simulink model "gm_uz_plantModel_pt1"  (R2020b)
settings: Solver=FixedStepAuto  StartTime=0.0  StopTime=20  RelTol=1e-3
libraries: dspsigops x11, hdlmdlgenlib x6
settings Model: Creator=ts  LastModifiedBy=ts
settings DataIOCC: LimitDataPoints=on  SaveOutput=off  SaveTime=off
settings OptimizationCC: BlockReduction=off  ConditionallyExecuteInputs=off  DefaultParameterBehavior=Inlined  LifeSpan=inf
settings DebuggingCC: AlgebraicLoopMsg=error  InheritedTsInSrcMsg=none  SingleTaskRateTransMsg=error  AllowSymbolicDim=off  StrictBusMsg=ErrorOnBusTreatedAsVector  SFUnexpectedBacktrackingDiag=warning  SFNoUnconditionalDefaultTransitionDiag=warning  SFExecutionAtInitializationDiag=none  ArithmeticOperatorsInVariantConditions=warning
settings HardwareCC: ProdBitPerPointer=32  ProdBitPerSizeT=32  ProdBitPerPtrDiffT=32  ProdLargestAtomicFloat=None  ProdIntDivRoundTo=Undefined  ProdEndianess=Unspecified  ProdWordSize=32  ProdHWDeviceType=ASIC/FPGA->ASIC/FPGA  ProdEqTarget=off
settings SFSimCC: SimUseLocalCustomCode=off  CustomCodeUndefinedFunction=UseInterfaceOnly
settings RTWCC: RTWUseLocalCustomCode=off
settings CodeAppCC: StateflowObjectComments=on
settings GRTTargetCC: TargetLangStandard=C89/C90 (ANSI)
settings ConfigComp: CovScope=ReferencedModels  CovMetricSettings=dw  CovSaveCumulativeToWorkspaceVar=on  CovSaveSingleToWorkspaceVar=on  CovExternalEMLEnable=off  CovSFcnEnable=off

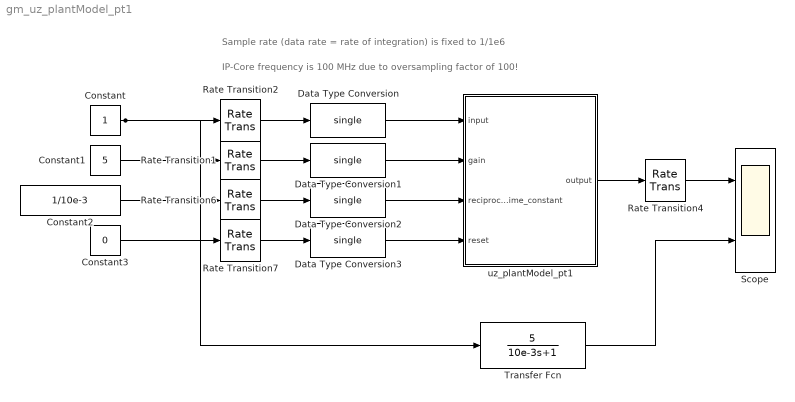
== system gm_uz_plantModel_pt1 ==
  note: Sample rate (data rate = rate of integration) is fixed to 1/1e6
  note: IP-Core frequency is 100 MHz due to oversampling factor of 100!
  Constant : Constant
  Constant1 : Constant  Value=5
  Constant2 : Constant  Value=1/10e-3
  Constant3 : Constant  Value=0
  Data Type Conversion{,1..3} (4 alike) : DataTypeConversion  OutDataTypeStr=single
  Rate Transition{1..2,6..7} (4 alike) : RateTransition  OutPortSampleTime=1/1e6
  Rate Transition4 : RateTransition
  Scope : Scope  NumInputPorts=2
  Transfer Fcn : TransferFcn  Numerator=[5]  Denominator=[10e-3 1]
  uz_plantModel_pt1 : Subsystem  TreatAsAtomicUnit=on
  wires:
  Constant3/1 -> Rate Transition7/1
  Constant2/1 -> Rate Transition6/1
  Constant1/1 -> Rate Transition1/1
  Rate Transition7/1 -> Data Type Conversion3/1
  Rate Transition6/1 -> Data Type Conversion2/1
  Rate Transition1/1 -> Data Type Conversion1/1
  Data Type Conversion3/1 -> uz_plantModel_pt1/4(reset)
  Data Type Conversion2/1 -> uz_plantModel_pt1/3(reciprocal_time_constant)
  Data Type Conversion1/1 -> uz_plantModel_pt1/2(gain)
  Data Type Conversion/1 -> uz_plantModel_pt1/1(input)
  Rate Transition2/1 -> Data Type Conversion/1
  Transfer Fcn/1 -> Scope/2
  Rate Transition4/1 -> Scope/1
  Constant/1 -> Transfer Fcn/1, Rate Transition2/1
  uz_plantModel_pt1/1(output) -> Rate Transition4/1

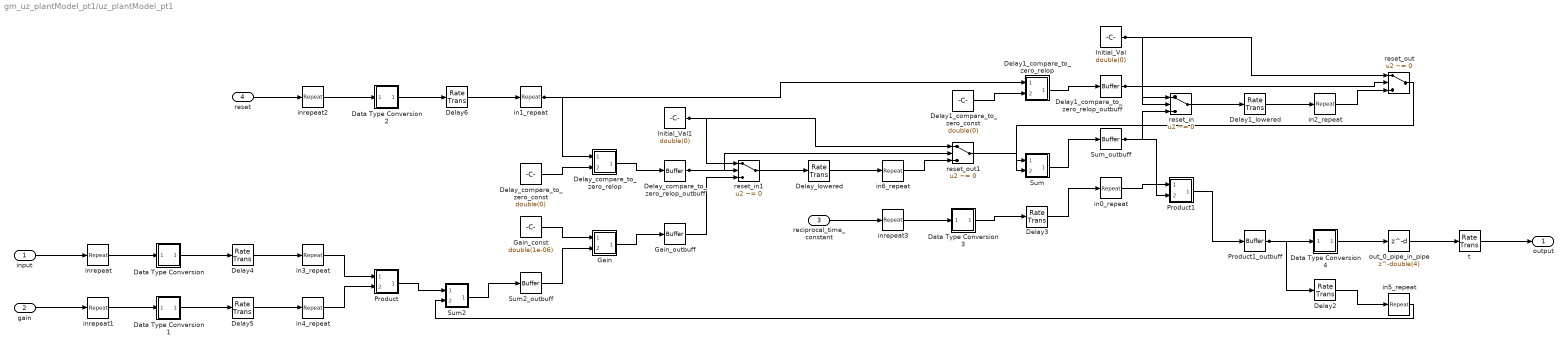
== system gm_uz_plantModel_pt1/uz_plantModel_pt1 ==
  input : Inport  OutDataTypeStr=single  PortDimensions=1  SampleTime=1e-06
  gain : Inport  Port=2  OutDataTypeStr=single  PortDimensions=1  SampleTime=1e-06
  reciprocal_time_constant : Inport  Port=3  OutDataTypeStr=single  PortDimensions=1  SampleTime=1e-06
  reset : Inport  Port=4  OutDataTypeStr=single  PortDimensions=1  SampleTime=1e-06
  Data Type Conversion : Subsystem
      mask Display: disp('NFP\nconv');
  Data Type Conversion1 : Subsystem
      mask Display: disp('NFP\nconv');
  Data Type Conversion2 : Subsystem
      mask Display: disp('NFP\nconv');
  Data Type Conversion3 : Subsystem
      mask Display: disp('NFP\nconv');
  Data Type Conversion4 : Subsystem
      mask Display: disp('NFP\nconv');
  Delay1_compare_to_zero_const : Constant  Value=double(0)  OutDataTypeStr=double  SampleTime=1e-08
  Delay1_compare_to_zero_relop : Subsystem
      mask Display: disp('NFP\nrelop');
  Delay1_compare_to_zero_relop_outbuff : hdlmdlgenlib/Buffer
      settings: SourceProductBaseCode=SL
  Delay1_lowered : RateTransition  OutPortSampleTimeOpt=Multiple of input port sample time  OutPortSampleTimeMultiple=100
  Delay{2..6} (5 alike) : RateTransition  OutPortSampleTimeOpt=Multiple of input port sample time  OutPortSampleTimeMultiple=100
  Delay_compare_to_zero_const : Constant  Value=double(0)  OutDataTypeStr=double  SampleTime=1e-08
  Delay_compare_to_zero_relop : Subsystem
      mask Display: disp('NFP\nrelop');
  Delay_compare_to_zero_relop_outbuff : hdlmdlgenlib/Buffer
      settings: SourceProductBaseCode=SL
  Delay_lowered : RateTransition  OutPortSampleTimeOpt=Multiple of input port sample time  OutPortSampleTimeMultiple=100
  Gain : Subsystem
      mask Display: disp('NFP\nmul');
  Gain_const : Constant  Value=double(1e-06)  OutDataTypeStr=double  SampleTime=1e-08
  Gain_outbuff : hdlmdlgenlib/Buffer
      settings: SourceProductBaseCode=SL
  Initial_Val : Constant  Value=double(0)  OutDataTypeStr=double  SampleTime=1e-08
  Initial_Val1 : Constant  Value=double(0)  OutDataTypeStr=double  SampleTime=1e-08
  Product : Subsystem
      mask Display: disp('NFP\nmul');
  Product1 : Subsystem
      mask Display: disp('NFP\nmul');
  Product1_outbuff : hdlmdlgenlib/Buffer
      settings: SourceProductBaseCode=SL
  Sum : Subsystem
      mask Display: disp('NFP\nadd');
  Sum2 : Subsystem
      mask Display: disp('NFP\nadd');
  Sum2_outbuff : hdlmdlgenlib/Buffer
      settings: SourceProductBaseCode=SL
  Sum_outbuff : hdlmdlgenlib/Buffer
      settings: SourceProductBaseCode=SL
  in0_repeat : dspsigops/Repeat  N=double(100)  RateOptions=Allow multirate processing  ic=0  mode=Unused parameter value
  in1_repeat : dspsigops/Repeat  N=double(100)  RateOptions=Allow multirate processing  ic=0  mode=Unused parameter value
  in2_repeat : dspsigops/Repeat  N=double(100)  RateOptions=Allow multirate processing  ic=0  mode=Unused parameter value
  in3_repeat : dspsigops/Repeat  N=double(100)  RateOptions=Allow multirate processing  ic=0  mode=Unused parameter value
  in4_repeat : dspsigops/Repeat  N=double(100)  RateOptions=Allow multirate processing  ic=0  mode=Unused parameter value
  in5_repeat : dspsigops/Repeat  N=double(100)  RateOptions=Allow multirate processing  ic=0  mode=Unused parameter value
  in6_repeat : dspsigops/Repeat  N=double(100)  RateOptions=Allow multirate processing  ic=0  mode=Unused parameter value
  inrepeat{,1..3} (4 alike) : dspsigops/Repeat  N=double(100)  RateOptions=Allow multirate processing  ic=0  mode=Unused parameter value
  out_0_pipe_in_pipe : Delay  DelayLength=double(4)  InitialCondition=0  SampleTime=1e-08
  reset_in : Switch  Criteria=u2 ~= 0  Threshold=double(0)  OutDataTypeStr=double  SampleTime=1e-08
  reset_in1 : Switch  Criteria=u2 ~= 0  Threshold=double(0)  OutDataTypeStr=double  SampleTime=1e-08
  reset_out : Switch  Criteria=u2 ~= 0  Threshold=double(0)  OutDataTypeStr=double  SampleTime=1e-08
  reset_out1 : Switch  Criteria=u2 ~= 0  Threshold=double(0)  OutDataTypeStr=double  SampleTime=1e-08
  t : RateTransition  OutPortSampleTimeOpt=Multiple of input port sample time  OutPortSampleTimeMultiple=100
  output : Outport
  wires:
  input/1 -> inrepeat/1
  gain/1 -> inrepeat1/1
  reciprocal_time_constant/1 -> inrepeat3/1
  reset/1 -> inrepeat2/1
  Delay4/1 -> in3_repeat/1
  Delay5/1 -> in4_repeat/1
  Delay6/1 -> in1_repeat/1
  Delay3/1 -> in0_repeat/1
  t/1 -> output/1
  Delay2/1 -> in5_repeat/1
  Delay1_lowered/1 -> in2_repeat/1
  Delay_lowered/1 -> in6_repeat/1
  Data Type Conversion/1(Out1) -> Delay4/1
  inrepeat/1 -> Data Type Conversion/1(In1)
  Data Type Conversion1/1(Out1) -> Delay5/1
  inrepeat1/1 -> Data Type Conversion1/1(In1)
  Data Type Conversion2/1(Out1) -> Delay6/1
  inrepeat2/1 -> Data Type Conversion2/1(In1)
  Data Type Conversion3/1(Out1) -> Delay3/1
  inrepeat3/1 -> Data Type Conversion3/1(In1)
  Product1_outbuff/1 -> Delay2/1, Data Type Conversion4/1(In1)
  reset_in/1 -> Delay1_lowered/1
  reset_in1/1 -> Delay_lowered/1
  in0_repeat/1 -> Product1/1(In1)
  in1_repeat/1 -> Delay_compare_to_zero_relop/1(In1), Delay1_compare_to_zero_relop/1(In1)
  in2_repeat/1 -> reset_out/3
  in3_repeat/1 -> Product/1(In1)
  in4_repeat/1 -> Product/2(In2)
  in5_repeat/1 -> Sum2/2(In2)
  in6_repeat/1 -> reset_out1/3
  Delay1_compare_to_zero_const/1 -> Delay1_compare_to_zero_relop/2(In2)
  reset_out/1 -> Sum/2(In2)
  Initial_Val/1 -> reset_out/1, reset_in/1
  Delay_compare_to_zero_const/1 -> Delay_compare_to_zero_relop/2(In2)
  Sum2_outbuff/1 -> Gain/2(In2)
  Gain_outbuff/1 -> reset_in1/3
  Initial_Val1/1 -> reset_out1/1, reset_in1/1
  reset_out1/1 -> Sum/1(In1)
  Sum_outbuff/1 -> Product1/2(In2), reset_in/3
  out_0_pipe_in_pipe/1 -> t/1
  Gain_const/1 -> Gain/1(In1)
  Delay1_compare_to_zero_relop/1(Out1) -> Delay1_compare_to_zero_relop_outbuff/1
  Delay_compare_to_zero_relop/1(Out1) -> Delay_compare_to_zero_relop_outbuff/1
  Product/1(Out1) -> Sum2/1(In1)
  Sum2/1(Out1) -> Sum2_outbuff/1
  Sum/1(Out1) -> Sum_outbuff/1
  Product1/1(Out1) -> Product1_outbuff/1
  Data Type Conversion4/1(Out1) -> out_0_pipe_in_pipe/1
  Gain/1(Out1) -> Gain_outbuff/1
  Delay1_compare_to_zero_relop_outbuff/1 -> reset_out/2, reset_in/2
  Delay_compare_to_zero_relop_outbuff/1 -> reset_out1/2, reset_in1/2

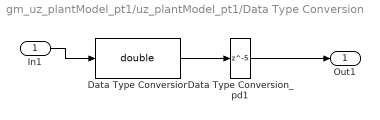
== system gm_uz_plantModel_pt1/uz_plantModel_pt1/Data Type Conversion ==
  In1 : Inport
  Data Type Conversion : DataTypeConversion  OutDataTypeStr=double  RndMeth=Nearest  SampleTime=1e-08
  Data Type Conversion_pd1 : Delay  DelayLength=5
  Out1 : Outport
  wires:
  In1/1 -> Data Type Conversion/1
  Data Type Conversion/1 -> Data Type Conversion_pd1/1
  Data Type Conversion_pd1/1 -> Out1/1

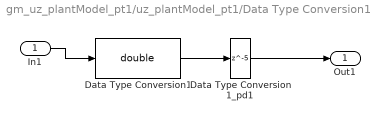
== system gm_uz_plantModel_pt1/uz_plantModel_pt1/Data Type Conversion1 ==
  In1 : Inport
  Data Type Conversion1 : DataTypeConversion  OutDataTypeStr=double  RndMeth=Nearest  SampleTime=1e-08
  Data Type Conversion1_pd1 : Delay  DelayLength=5
  Out1 : Outport
  wires:
  In1/1 -> Data Type Conversion1/1
  Data Type Conversion1/1 -> Data Type Conversion1_pd1/1
  Data Type Conversion1_pd1/1 -> Out1/1

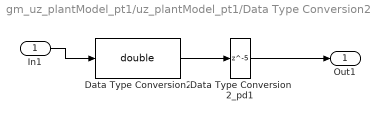
== system gm_uz_plantModel_pt1/uz_plantModel_pt1/Data Type Conversion2 ==
  In1 : Inport
  Data Type Conversion2 : DataTypeConversion  OutDataTypeStr=double  RndMeth=Nearest  SampleTime=1e-08
  Data Type Conversion2_pd1 : Delay  DelayLength=5
  Out1 : Outport
  wires:
  In1/1 -> Data Type Conversion2/1
  Data Type Conversion2/1 -> Data Type Conversion2_pd1/1
  Data Type Conversion2_pd1/1 -> Out1/1

== system gm_uz_plantModel_pt1/uz_plantModel_pt1/Data Type Conversion3 ==
  In1 : Inport
  Data Type Conversion3 : DataTypeConversion  OutDataTypeStr=double  RndMeth=Nearest  SampleTime=1e-08
  Data Type Conversion3_pd1 : Delay  DelayLength=5
  Out1 : Outport
  wires:
  In1/1 -> Data Type Conversion3/1
  Data Type Conversion3/1 -> Data Type Conversion3_pd1/1
  Data Type Conversion3_pd1/1 -> Out1/1

== system gm_uz_plantModel_pt1/uz_plantModel_pt1/Data Type Conversion4 ==
  In1 : Inport
  Data Type Conversion4 : DataTypeConversion  OutDataTypeStr=single  RndMeth=Nearest  SampleTime=1e-08
  Data Type Conversion4_pd1 : Delay  DelayLength=6
  Out1 : Outport
  wires:
  In1/1 -> Data Type Conversion4/1
  Data Type Conversion4/1 -> Data Type Conversion4_pd1/1
  Data Type Conversion4_pd1/1 -> Out1/1

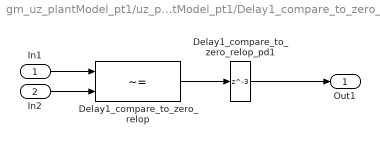
== system gm_uz_plantModel_pt1/uz_plantModel_pt1/Delay1_compare_to_zero_relop ==
  In1 : Inport
  In2 : Inport  Port=2
  Delay1_compare_to_zero_relop : RelationalOperator  Operator=~=  OutDataTypeStr=boolean  SampleTime=1e-08  RndMeth=Nearest  InputSameDT=on
  Delay1_compare_to_zero_relop_pd1 : Delay  DelayLength=3
  Out1 : Outport
  wires:
  In1/1 -> Delay1_compare_to_zero_relop/1
  In2/1 -> Delay1_compare_to_zero_relop/2
  Delay1_compare_to_zero_relop/1 -> Delay1_compare_to_zero_relop_pd1/1
  Delay1_compare_to_zero_relop_pd1/1 -> Out1/1

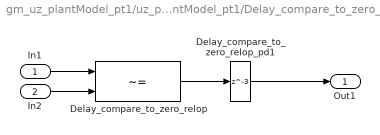
== system gm_uz_plantModel_pt1/uz_plantModel_pt1/Delay_compare_to_zero_relop ==
  In1 : Inport
  In2 : Inport  Port=2
  Delay_compare_to_zero_relop : RelationalOperator  Operator=~=  OutDataTypeStr=boolean  SampleTime=1e-08  RndMeth=Nearest  InputSameDT=on
  Delay_compare_to_zero_relop_pd1 : Delay  DelayLength=3
  Out1 : Outport
  wires:
  In1/1 -> Delay_compare_to_zero_relop/1
  In2/1 -> Delay_compare_to_zero_relop/2
  Delay_compare_to_zero_relop/1 -> Delay_compare_to_zero_relop_pd1/1
  Delay_compare_to_zero_relop_pd1/1 -> Out1/1

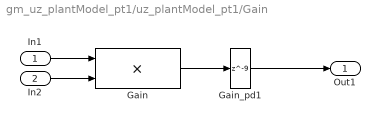
== system gm_uz_plantModel_pt1/uz_plantModel_pt1/Gain ==
  In1 : Inport
  In2 : Inport  Port=2
  Gain : Product  Inputs=**  OutDataTypeStr=double  SampleTime=1e-08
  Gain_pd1 : Delay  DelayLength=9
  Out1 : Outport
  wires:
  In1/1 -> Gain/1
  In2/1 -> Gain/2
  Gain/1 -> Gain_pd1/1
  Gain_pd1/1 -> Out1/1

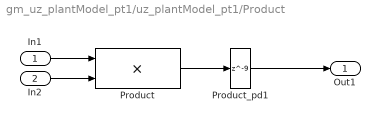
== system gm_uz_plantModel_pt1/uz_plantModel_pt1/Product ==
  In1 : Inport
  In2 : Inport  Port=2
  Product : Product  Inputs=**  OutDataTypeStr=double  SampleTime=1e-08
  Product_pd1 : Delay  DelayLength=9
  Out1 : Outport
  wires:
  In1/1 -> Product/1
  In2/1 -> Product/2
  Product/1 -> Product_pd1/1
  Product_pd1/1 -> Out1/1

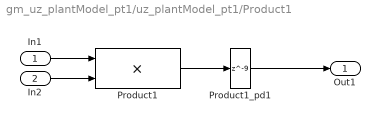
== system gm_uz_plantModel_pt1/uz_plantModel_pt1/Product1 ==
  In1 : Inport
  In2 : Inport  Port=2
  Product1 : Product  Inputs=**  OutDataTypeStr=double  SampleTime=1e-08
  Product1_pd1 : Delay  DelayLength=9
  Out1 : Outport
  wires:
  In1/1 -> Product1/1
  In2/1 -> Product1/2
  Product1/1 -> Product1_pd1/1
  Product1_pd1/1 -> Out1/1

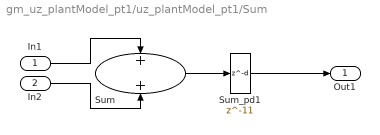
== system gm_uz_plantModel_pt1/uz_plantModel_pt1/Sum ==
  In1 : Inport
  In2 : Inport  Port=2
  Sum : Sum  OutDataTypeStr=double  SampleTime=1e-08
  Sum_pd1 : Delay  DelayLength=11
  Out1 : Outport
  wires:
  In1/1 -> Sum/1
  In2/1 -> Sum/2
  Sum/1 -> Sum_pd1/1
  Sum_pd1/1 -> Out1/1

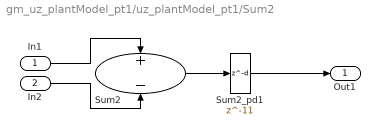
== system gm_uz_plantModel_pt1/uz_plantModel_pt1/Sum2 ==
  In1 : Inport
  In2 : Inport  Port=2
  Sum2 : Sum  Inputs=+-  OutDataTypeStr=double  SampleTime=1e-08
  Sum2_pd1 : Delay  DelayLength=11
  Out1 : Outport
  wires:
  In1/1 -> Sum2/1
  In2/1 -> Sum2/2
  Sum2/1 -> Sum2_pd1/1
  Sum2_pd1/1 -> Out1/1
